simulink model "project3_v1"  (R2021a)
settings: Solver=VariableStepAuto  StartTime=0.0  StopTime=30  RelTol=1e-3
libraries: hdlBasic x25, xbsIndex_r4 x1
settings Model: Creator=caval  LastModifiedBy=hl116

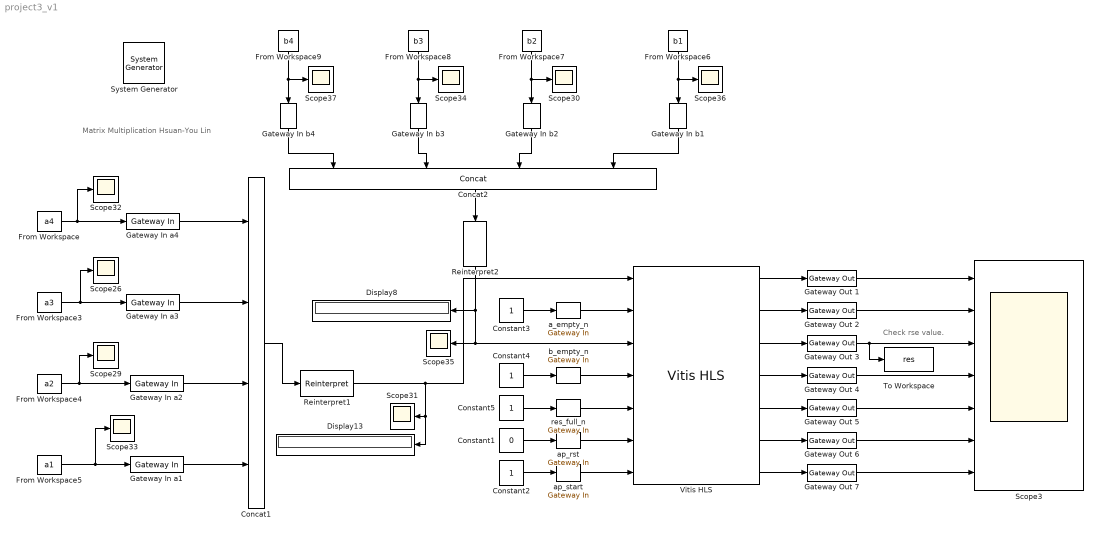
== system project3_v1 ==
  note: Matrix Multiplication
      | Hsuan-You Lin
  note: Check rse value.
  " System Generator" : xbsIndex_r4/ System Generator  Tag=genX  xilinxfamily=zynq  part=xc7z020  speed=-1  package=clg484  synthesis_tool=Vivado  clock_wrapper=Clock Enables  directory=./netlist  proj_type=Vivado  Synth_file=Vivado Synthesis Defaults  Impl_file=Vivado Implementation Defaults  testbench=off  simulink_period=1  sysclk_period=10  dcm_input_clock_period=10  incr_netlist=off  trim_vbits=Everywhere in SubSystem  dbl_ovrd=According to Block Masks  core_generation=According to Block Masks  run_coregen=off  deprecated_control=off  eval_field=0  block_type=sysgen
  Concat1 : hdlBasic/Concat  num_inputs=4  XmcBlockStatus=1  maskContainerNames=group1  block_type=concat  block_config=sysgen:Concat_config
  Concat2 : hdlBasic/Concat  num_inputs=4  XmcBlockStatus=1  maskContainerNames=group1  block_type=concat  block_config=sysgen:Concat_config
  Constant1 : Constant  Value=0
  Constant{2..5} (4 alike) : Constant
  Display13 : Display
      settings: Format=hex (Stored Integer)
  Display8 : Display
      settings: Format=hex (Stored Integer)
  From Workspace : FromWorkspace  VariableName=a4
  From Workspace3 : FromWorkspace  VariableName=a3
  From Workspace4 : FromWorkspace  VariableName=a2
  From Workspace5 : FromWorkspace  VariableName=a1
  From Workspace6 : FromWorkspace  VariableName=b1
  From Workspace7 : FromWorkspace  VariableName=b2
  From Workspace8 : FromWorkspace  VariableName=b3
  From Workspace9 : FromWorkspace  VariableName=b4
  Gateway In a{1..4} (4 alike) : hdlBasic/Gateway In  gui_display_data_type=Fixed-point  arith_type=Unsigned  n_bits=16  bin_pt=0  preci_type=Single  exp_width=8  frac_width=24  rows=1  columns=1  quantization="Round  (unbiased: +/- Inf)"  overflow=Saturate  period=1  UseAsADC=off  ADCChannel='1'  interface=None  automatic_assignment=on  address_offset=hex2dec('00')  intf_name=''  intf_description=''  default_value=0  timing_constraint=None  locs_specified=off  LOCs={}  io_standard={}  inherit_from_input=off  hdl_port=on  XmcBlockStatus=1  maskContainerNames=group4  block_type=gatewayin  block_config=sysgen:gateway_in_config  block_width_w=590  block_height_w=620  block_width=640  block_height=850
  Gateway In b{1..4} (4 alike) : hdlBasic/Gateway In  gui_display_data_type=Fixed-point  arith_type=Unsigned  n_bits=16  bin_pt=0  preci_type=Single  exp_width=8  frac_width=24  rows=1  columns=1  quantization="Round  (unbiased: +/- Inf)"  overflow=Saturate  period=1  UseAsADC=off  ADCChannel='1'  interface=None  automatic_assignment=on  address_offset=hex2dec('00')  intf_name=''  intf_description=''  default_value=0  timing_constraint=None  locs_specified=off  LOCs={}  io_standard={}  inherit_from_input=off  hdl_port=on  XmcBlockStatus=1  maskContainerNames=group4  block_type=gatewayin  block_config=sysgen:gateway_in_config  block_width_w=590  block_height_w=620  block_width=640  block_height=850
  Gateway Out {1..7} (7 alike) : hdlBasic/Gateway Out  inherit_from_input=on  hdl_port=on  rows=1  columns=1  UseAsDAC=off  DACChannel='1'  interface=None  automatic_assignment=on  address_offset=hex2dec('00')  intf_name=''  intf_description='Output_R'  timing_constraint=None  locs_specified=off  LOCs={}  io_standard={}  XmcBlockStatus=1  maskContainerNames=group4  block_type=gatewayout  block_config=sysgen:gateway_out_config  block_width_w=590  block_height_w=620  block_width=620  block_height=750
  Reinterpret1 : hdlBasic/Reinterpret  force_arith_type=on  arith_type="Signed  (2's comp)"  force_bin_pt=off  bin_pt=0  XmcBlockStatus=1  maskContainerNames=group1  block_type=reinterpret  block_config=sysgen:Reinterpret_config
  Reinterpret2 : hdlBasic/Reinterpret  force_arith_type=on  arith_type="Signed  (2's comp)"  force_bin_pt=off  bin_pt=0  XmcBlockStatus=1  maskContainerNames=group1  block_type=reinterpret  block_config=sysgen:Reinterpret_config
  Scope{26,29..37} (10 alike) : Scope
  Scope3 : Scope  NumInputPorts=7
  To Workspace : ToWorkspace  VariableName=res  SaveFormat=Timeseries  SampleTime=-1
      settings: Save2DSignal=2-D array (concatenate along first dimension)
  Vitis HLS : hdlBasic/Vitis HLS  anytable='.\Project3_v1_hls\solution4_Final'  fast_sim=off  display_datatype=off  rate_propagation_method=Simulink system period  model_file_path=''  latency=1  block_type=vitis_hls
      settings: infoedit=This block allows including C,C++ and SystemC source files in System Generator for DSP designs.
  "a_empty_n " : hdlBasic/Gateway In  gui_display_data_type=Boolean  arith_type=Boolean  n_bits=16  bin_pt=0  preci_type=Single  exp_width=8  frac_width=24  rows=1  columns=1  quantization="Round  (unbiased: +/- Inf)"  overflow=Saturate  period=1  UseAsADC=off  ADCChannel='1'  interface=None  automatic_assignment=on  address_offset=hex2dec('00')  intf_name=''  intf_description='Input_A'  default_value=0  timing_constraint=None  locs_specified=off  LOCs={}  io_standard={}  inherit_from_input=off  hdl_port=on  XmcBlockStatus=1  maskContainerNames=group4  block_type=gatewayin  block_config=sysgen:gateway_in_config  block_width_w=590  block_height_w=620  block_width=640  block_height=850
  ap_rst : hdlBasic/Gateway In  gui_display_data_type=Boolean  arith_type=Boolean  n_bits=16  bin_pt=0  preci_type=Single  exp_width=8  frac_width=24  rows=1  columns=1  quantization="Round  (unbiased: +/- Inf)"  overflow=Saturate  period=1  UseAsADC=off  ADCChannel='1'  interface=None  automatic_assignment=on  address_offset=hex2dec('00')  intf_name=''  intf_description='Input_A'  default_value=0  timing_constraint=None  locs_specified=off  LOCs={}  io_standard={}  inherit_from_input=off  hdl_port=on  XmcBlockStatus=1  maskContainerNames=group4  block_type=gatewayin  block_config=sysgen:gateway_in_config  block_width_w=590  block_height_w=620  block_width=640  block_height=850
  "ap_start " : hdlBasic/Gateway In  gui_display_data_type=Boolean  arith_type=Boolean  n_bits=16  bin_pt=0  preci_type=Single  exp_width=8  frac_width=24  rows=1  columns=1  quantization="Round  (unbiased: +/- Inf)"  overflow=Saturate  period=1  UseAsADC=off  ADCChannel='1'  interface=None  automatic_assignment=on  address_offset=hex2dec('00')  intf_name=''  intf_description='Input_A'  default_value=0  timing_constraint=None  locs_specified=off  LOCs={}  io_standard={}  inherit_from_input=off  hdl_port=on  XmcBlockStatus=1  maskContainerNames=group4  block_type=gatewayin  block_config=sysgen:gateway_in_config  block_width_w=590  block_height_w=620  block_width=640  block_height=850
  b_empty_n : hdlBasic/Gateway In  gui_display_data_type=Boolean  arith_type=Boolean  n_bits=16  bin_pt=0  preci_type=Single  exp_width=8  frac_width=24  rows=1  columns=1  quantization="Round  (unbiased: +/- Inf)"  overflow=Saturate  period=1  UseAsADC=off  ADCChannel='1'  interface=None  automatic_assignment=on  address_offset=hex2dec('00')  intf_name=''  intf_description='Input_A'  default_value=0  timing_constraint=None  locs_specified=off  LOCs={}  io_standard={}  inherit_from_input=off  hdl_port=on  XmcBlockStatus=1  maskContainerNames=group4  block_type=gatewayin  block_config=sysgen:gateway_in_config  block_width_w=590  block_height_w=620  block_width=640  block_height=850
  res_full_n : hdlBasic/Gateway In  gui_display_data_type=Boolean  arith_type=Boolean  n_bits=16  bin_pt=0  preci_type=Single  exp_width=8  frac_width=24  rows=1  columns=1  quantization="Round  (unbiased: +/- Inf)"  overflow=Saturate  period=1  UseAsADC=off  ADCChannel='1'  interface=None  automatic_assignment=on  address_offset=hex2dec('00')  intf_name=''  intf_description='Input_A'  default_value=0  timing_constraint=None  locs_specified=off  LOCs={}  io_standard={}  inherit_from_input=off  hdl_port=on  XmcBlockStatus=1  maskContainerNames=group4  block_type=gatewayin  block_config=sysgen:gateway_in_config  block_width_w=590  block_height_w=620  block_width=640  block_height=850
  wires:
  Constant1/1 -> ap_rst/1
  Constant2/1 -> "ap_start "/1
  From Workspace4/1 -> Scope29/1, Gateway In a2/1
  From Workspace5/1 -> Scope33/1, Gateway In a1/1
  Gateway In a4/1 -> Concat1/1
  Gateway In a3/1 -> Concat1/2
  Gateway In a2/1 -> Concat1/3
  Gateway In a1/1 -> Concat1/4
  From Workspace3/1 -> Scope26/1, Gateway In a3/1
  Reinterpret1/1 -> Display13/1, Scope31/1, Vitis HLS/1
  Concat1/1 -> Reinterpret1/1
  From Workspace/1 -> Gateway In a4/1, Scope32/1
  From Workspace8/1 -> Gateway In b3/1, Scope34/1
  From Workspace7/1 -> Scope30/1, Gateway In b2/1
  Concat2/1 -> Reinterpret2/1
  From Workspace6/1 -> Gateway In b1/1, Scope36/1
  From Workspace9/1 -> Scope37/1, Gateway In b4/1
  Gateway In b4/1 -> Concat2/1
  Gateway In b3/1 -> Concat2/2
  Gateway In b2/1 -> Concat2/3
  Gateway In b1/1 -> Concat2/4
  Constant3/1 -> "a_empty_n "/1
  Constant4/1 -> b_empty_n/1
  Constant5/1 -> res_full_n/1
  Vitis HLS/2 -> Gateway Out 2/1
  Vitis HLS/1 -> Gateway Out 1/1
  Vitis HLS/3 -> Gateway Out 3/1
  Vitis HLS/4 -> Gateway Out 4/1
  Vitis HLS/5 -> Gateway Out 5/1
  Vitis HLS/7 -> Gateway Out 7/1
  Gateway Out 3/1 -> To Workspace/1, Scope3/3
  Gateway Out 2/1 -> Scope3/2
  Gateway Out 1/1 -> Scope3/1
  Gateway Out 4/1 -> Scope3/4
  Gateway Out 5/1 -> Scope3/5
  Gateway Out 7/1 -> Scope3/7
  Vitis HLS/6 -> Gateway Out 6/1
  Gateway Out 6/1 -> Scope3/6
  "a_empty_n "/1 -> Vitis HLS/2
  b_empty_n/1 -> Vitis HLS/4
  res_full_n/1 -> Vitis HLS/5
  ap_rst/1 -> Vitis HLS/6
  "ap_start "/1 -> Vitis HLS/7
  Reinterpret2/1 -> Display8/1, Scope35/1, Vitis HLS/3
